simulink model "Servo_Observer"  (R2021b)
settings: Solver=ode45  StartTime=0.0  StopTime=1  RelTol=1e-3
values from neighbouring files (symbols this model uses):
  KI = K(4)    [Project.m]
  Kp = K(1:3)    [Project.m]
  L = IQ * ([Cz ; Cz*G ; Cz*(G^2)]^(-1))*[0 ; 0 ; 1]    [Project.m]
  Ts = 0.02    [Project.m]
undefined symbols (not defined in the file or in its folder): Cz, G, H
settings Model: Creator=Amir  LastModifiedBy=Amir

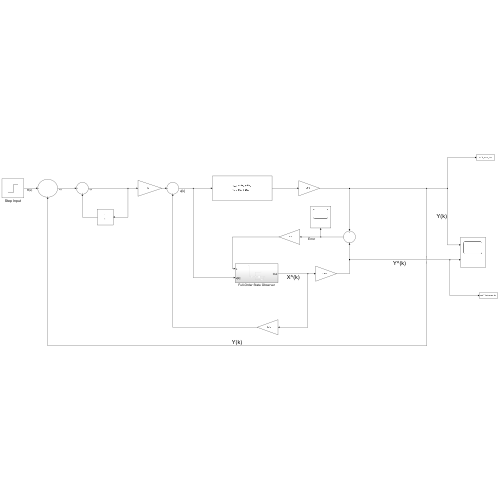
[thumbnail: Simulink's stored preview of the top-level diagram]
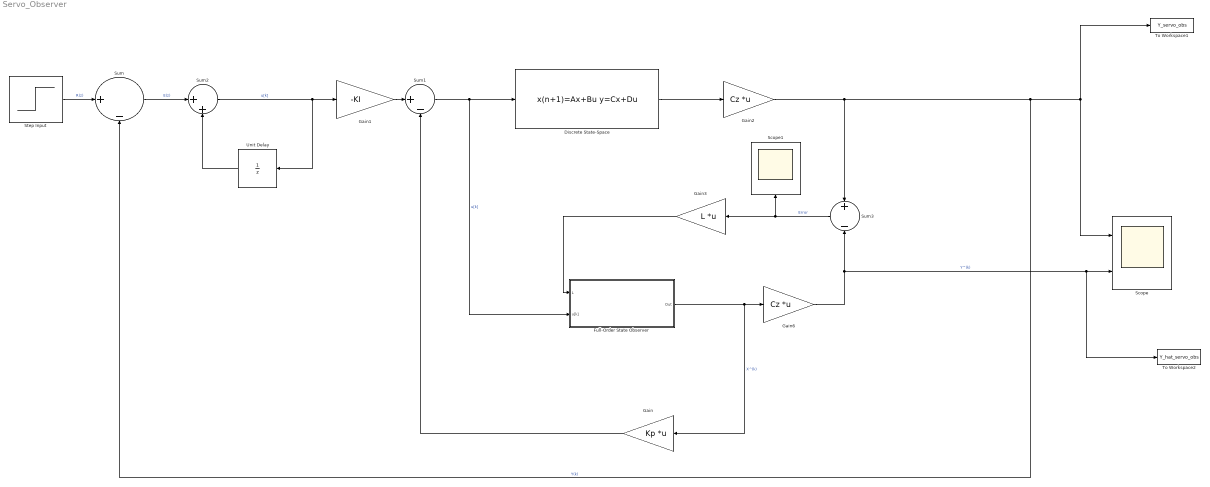
== system Servo_Observer ==
  Discrete State-Space : DiscreteStateSpace  A=G  B=H  C=eye(3)  D=zeros(3,1)  SampleTime=Ts
  Full-Order State Observer : Subsystem
  Gain : Gain  Gain=Kp  Multiplication=Matrix(K*u)
  Gain1 : Gain  Gain=-KI
  Gain2 : Gain  Gain=Cz  Multiplication=Matrix(K*u)
  Gain3 : Gain  Gain=L  Multiplication=Matrix(K*u)
  Gain6 : Gain  Gain=Cz  Multiplication=Matrix(K*u)
  Scope : Scope  NumInputPorts=2
  Scope1 : Scope
  Step Input : Step  Time=0  After=0.01  SampleTime=0
  Sum : Sum  Inputs=|+-
  Sum1 : Sum  Inputs=|+-
  Sum2 : Sum  Inputs=|++
  Sum3 : Sum  Inputs=+|-
  To Workspace1 : ToWorkspace  VariableName=Y_servo_obs  SaveFormat=Timeseries  SampleTime=-1
  To Workspace2 : ToWorkspace  VariableName=Y_hat_servo_obs  SaveFormat=Timeseries  SampleTime=-1
  Unit Delay : UnitDelay  SampleTime=-1  HasFrameUpgradeWarning=on
  wires:
  Discrete State-Space/1 -> Gain2/1
  Step Input/1 -> Sum/1  "R(z)"
  Sum1/1 -> Full-Order State Observer/2(u[k]), Discrete State-Space/1  "u[k]"
  Gain1/1 -> Sum1/1
  Sum2/1 -> Gain1/1, Unit Delay/1  "u[k]"
  Sum/1 -> Sum2/1  "E(z)"
  Gain2/1 -> Sum3/1, To Workspace1/1, Scope/1, Sum/2  "Y(k)"
  Unit Delay/1 -> Sum2/2
  Sum3/1 -> Gain3/1, Scope1/1  "Error"
  Gain6/1 -> To Workspace2/1, Scope/2, Sum3/2  "Y^(k)"
  Gain/1 -> Sum1/2
  Full-Order State Observer/1(Out) -> Gain/1, Gain6/1  "X^(k)"
  Gain3/1 -> Full-Order State Observer/1(L)

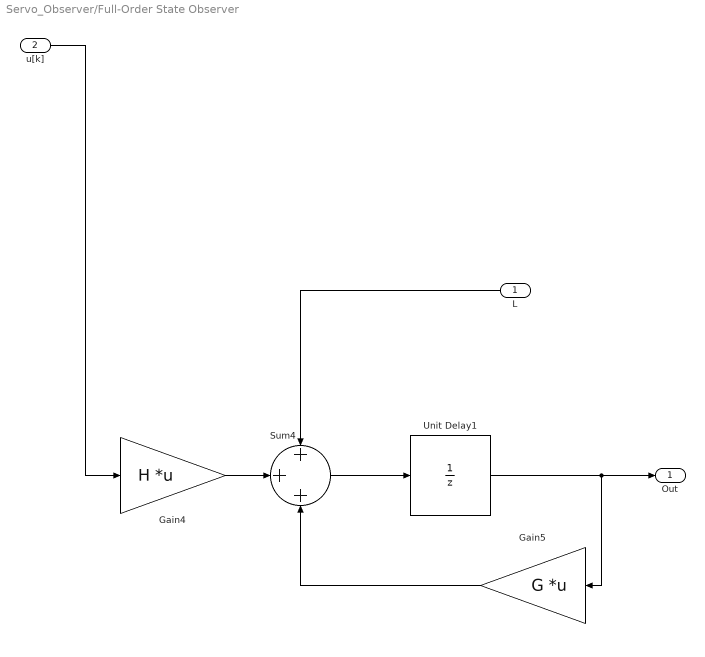
== system Servo_Observer/Full-Order State Observer ==
  L : Inport
  u[k] : Inport  Port=2
  Gain4 : Gain  Gain=H  Multiplication=Matrix(K*u)
  Gain5 : Gain  Gain=G  Multiplication=Matrix(K*u)
  Sum4 : Sum  Inputs=+++
  Unit Delay1 : UnitDelay  SampleTime=-1  HasFrameUpgradeWarning=on
  Out : Outport
  wires:
  Unit Delay1/1 -> Out/1, Gain5/1
  Gain5/1 -> Sum4/3
  L/1 -> Sum4/1
  Gain4/1 -> Sum4/2
  Sum4/1 -> Unit Delay1/1
  u[k]/1 -> Gain4/1
